simulink model "carcomplexsimulink_sim"  (R2025b)
settings: Solver=VariableStepAuto  StartTime=0.0  StopTime=10.0  RelTol=1e-3
settings Model: Creator=sprinkle  LastModifiedBy=sprinkle

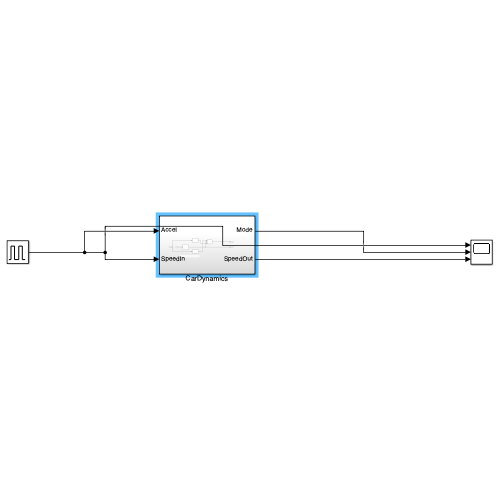
[thumbnail: Simulink's stored preview of the top-level diagram]
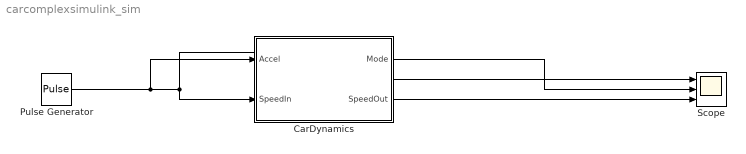
== system carcomplexsimulink_sim ==
  CarDynamics : Subsystem
  Pulse Generator : DiscretePulseGenerator  PulseType=Time based  Amplitude=1.5  Period=3  PulseWidth=50
  Scope : Scope  NumInputPorts=3
      settings: ActiveDisplayYMinimum=-1.68639300553092  ActiveDisplayYMaximum=1.8219726990969081
  wires:
  Pulse Generator/1 -> CarDynamics/1(Accel), CarDynamics/2(SpeedIn), Scope/1
  CarDynamics/1(Mode) -> Scope/2
  CarDynamics/2(SpeedOut) -> Scope/3

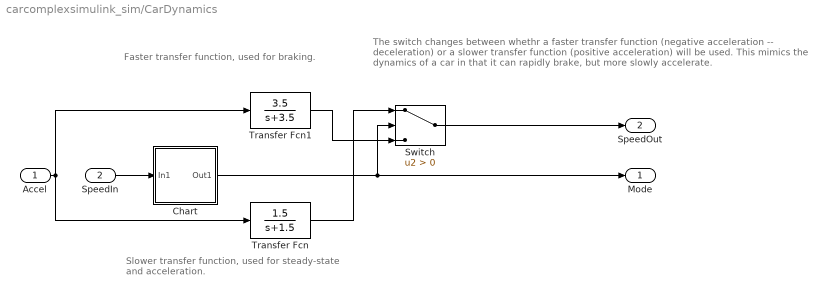
== system carcomplexsimulink_sim/CarDynamics ==
  note: The switch changes between whethr a faster transfer function (negative acceleration -- deceleration) or a slower transfer function (positive acceleration) will be used. This mimics the dynamics of a car in that it can rapidly brake, but more slowly accelerate.
  note: Faster transfer function, used for braking.
  note: Slower transfer function, used for steady-state and acceleration.
  Accel : Inport
  SpeedIn : Inport  Port=2
  Chart : Stateflow chart  TreatAsAtomicUnit=on
  Switch : Switch  Criteria=u2 > Threshold  SaturateOnIntegerOverflow=off  InputSameDT=off
  Transfer Fcn : TransferFcn  Numerator=[1.5]  Denominator=[1 1.5]
  Transfer Fcn1 : TransferFcn  Numerator=[3.5]  Denominator=[1 3.5]
  Mode : Outport
  SpeedOut : Outport  Port=2
  wires:
  Accel/1 -> Transfer Fcn/1, Transfer Fcn1/1
  SpeedIn/1 -> Chart/1(In1)
  Transfer Fcn1/1 -> Switch/3
  Switch/1 -> SpeedOut/1
  Transfer Fcn/1 -> Switch/1
  Chart/1(Out1) -> Mode/1, Switch/2

== stateflow chart carcomplexsimulink_sim/CarDynamics/Chart ==
  state Default
    entry: Out1=1;
  state Slowing
    entry: Out1=-1;
  (default) -> Default
  Slowing -> Default : [In1 > 0]
  Default -> Slowing : [In1 < 0.2]
  data: In1 input; Out1 output
